simulink model "YAW_tf_first_order"  (R2023b)
settings: Solver=VariableStepAuto  StartTime=0.0  StopTime=t(end)  RelTol=1e-3
settings Model: Creator=franc  LastModifiedBy=franc

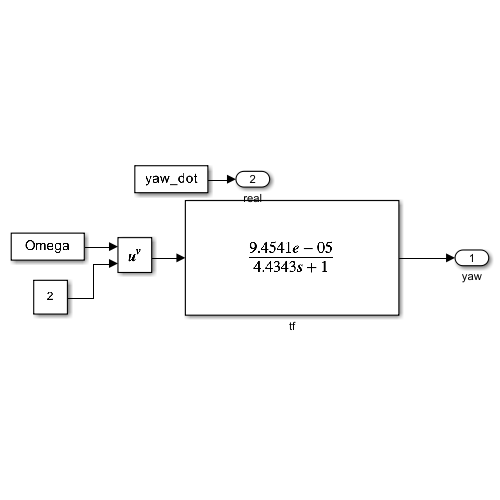
[thumbnail: Simulink's stored preview of the top-level diagram]
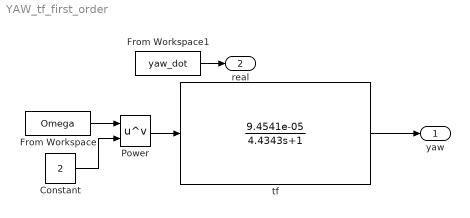
== system YAW_tf_first_order ==
  Constant : Constant  Value=2
  From Workspace : FromWorkspace  VariableName=Omega  SampleTime=0.002
  From Workspace1 : FromWorkspace  VariableName=yaw_dot
  Power : Math  Operator=pow
  tf : TransferFcn  Numerator=9.4541e-05  Denominator=[4.4343 1]
  yaw : Outport
  real : Outport  Port=2
  wires:
  Power/1 -> tf/1
  tf/1 -> yaw/1
  Constant/1 -> Power/2
  From Workspace1/1 -> real/1
  From Workspace/1 -> Power/1
